simulink model "Exercise1"  (R2024b)
settings: Solver=VariableStepAuto  StartTime=0.0  StopTime=seconds(missionduration)  FixedStep=1  MaxStep=5  RelTol=0.5e-5  AbsTol=1e-5
undefined symbols (not defined in the file): IAU, juliandate, missionstartdate, targetAmazon, targetNO
libraries: aerolibtransform2 x3, aerolibguid x2, aerolibsatdyn x1, aerolibutil x1
settings Model: Creator=The MathWorks, Inc.  LastModifiedBy=jbrault
settings SolverCC: MaxConsecutiveMinStep=10  AutoInsertRateTranBlk=on  DecoupledContinuousIntegration=on  MinimalZcImpactIntegration=on  MaxZcPerStep=1
settings DataIOCC: DatasetSignalFormat=timetable  LoggingIntervals=[0, inf]
settings DebuggingCC: ReadBeforeWriteMsg=DisableAll  WriteAfterWriteMsg=DisableAll  WriteAfterReadMsg=DisableAll  MultiTaskDSMMsg=none  UnconnectedInputMsg=warning  UnconnectedOutputMsg=warning  UnconnectedLineMsg=warning
settings ModelReferenceCC: UpdateModelReferenceTargets=IfOutOfDate  EnableRefExpFcnMdlSchedulingChecks=on
settings SFSimCC: SFSimEcho=off
settings RTWCC: GPUComputeCapability=3.5  DLArmComputeVersion=19.05

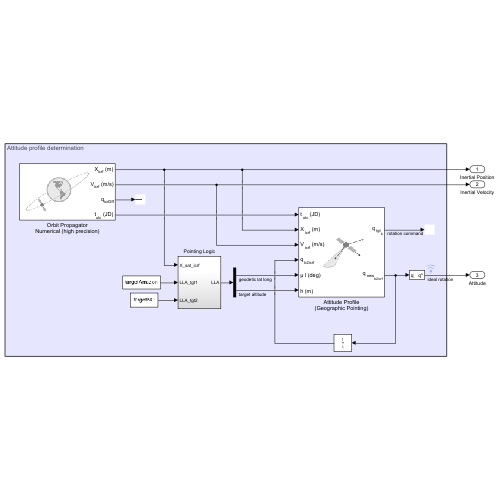
[thumbnail: Simulink's stored preview of the top-level diagram]
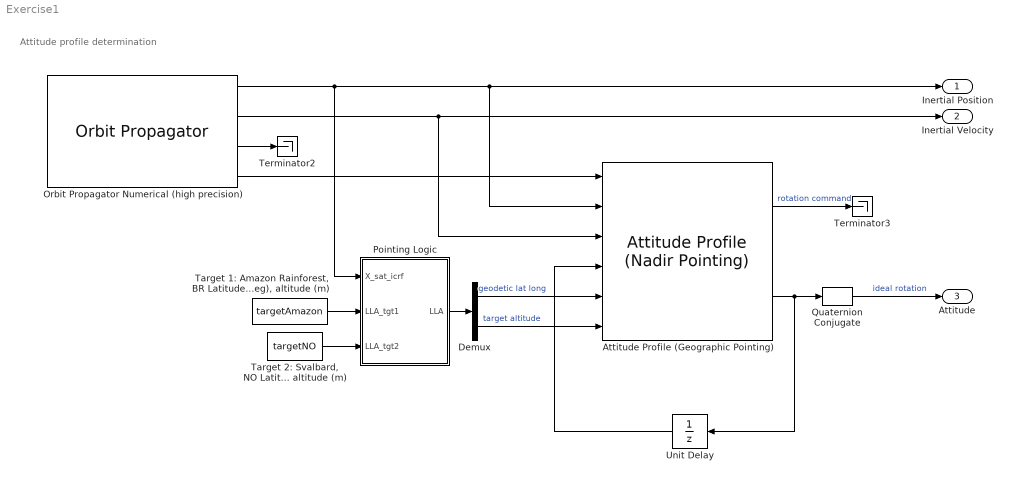
== system Exercise1 ==
  note: Attitude profile determination
  Attitude Profile (Geographic Pointing) : aerolibsatdyn/Attitude Profile (Nadir Pointing)  outputError=on  outputFinalAttitude=on  portFrame=ICRF  pointingMode=Point at LatLonAlt  celestialTarget=Sun  tunablePointing=off  primaryAlignmentSrc=Dialog  primaryAlignment=[0 0 1]  secondaryAlignmentSrc=Dialog  secondaryAlignment=[1 0 0]  constraintFrame=LVLH  primaryConstraintSrc=Dialog  primaryConstraint=[1 0 0]  secondaryConstraintSrc=Dialog  secondaryConstraint=[0 1 0]
  Demux : Demux  Outputs=[2 1]
  Orbit Propagator Numerical (high precision) : OrbitPropagator  propagator=Numerical (high precision)  startDate=juliandate(missionstartdate)  semiMajorAxis=7200000  eccentricity=0.05  inclination=70  raan=215  argPeriapsis=0  trueAnomaly=200  inertialPosition=[3649700.0 3308200.0 -4676600.0]  inertialVelocity=[-2750.8 6666.4 2573.4]  fixedPosition=[-4142689.0 -2676864.7 -4669861.6]  fixedVelocity=[1452.7 -6720.7 2568.1]  customR=3396200  customMu=4.305e13  customJ2=1.0826269e-03  customOmega=4.06125949e-3  outputTransform=on
  Pointing Logic : Subsystem
  Quaternion Conjugate : aerolibutil/Quaternion Conjugate
  "Target 1: Amazon Rainforest, BR Latitude (deg), Longitude (deg), altitude (m)" : Constant  Value=targetAmazon
  "Target 2: Svalbard, NO Latitude (deg), Longitude (deg), altitude (m)" : Constant  Value=targetNO
  Terminator2 : Terminator
  Terminator3 : Terminator
  Unit Delay : UnitDelay  InitialCondition=[1 0 0 0]  SampleTime=-1  HasFrameUpgradeWarning=on
  Inertial Position : Outport
  Inertial Velocity : Outport  Port=2
  Attitude : Outport  Port=3
  wires:
  Orbit Propagator Numerical (high precision)/2 -> Inertial Velocity/1, Attitude Profile (Geographic Pointing)/3
  Orbit Propagator Numerical (high precision)/1 -> Pointing Logic/1(X_sat_icrf), Inertial Position/1, Attitude Profile (Geographic Pointing)/2
  Demux/1 -> Attitude Profile (Geographic Pointing)/5  "geodetic lat long"
  Demux/2 -> Attitude Profile (Geographic Pointing)/6  "target altitude"
  Pointing Logic/1(LLA) -> Demux/1
  "Target 1: Amazon Rainforest, BR Latitude (deg), Longitude (deg), altitude (m)"/1 -> Pointing Logic/2(LLA_tgt1)
  "Target 2: Svalbard, NO Latitude (deg), Longitude (deg), altitude (m)"/1 -> Pointing Logic/3(LLA_tgt2)
  Attitude Profile (Geographic Pointing)/2 -> Quaternion Conjugate/1, Unit Delay/1
  Orbit Propagator Numerical (high precision)/3 -> Terminator2/1
  Orbit Propagator Numerical (high precision)/4 -> Attitude Profile (Geographic Pointing)/1
  Attitude Profile (Geographic Pointing)/1 -> Terminator3/1  "rotation command"
  Unit Delay/1 -> Attitude Profile (Geographic Pointing)/4
  Quaternion Conjugate/1 -> Attitude/1  "ideal rotation"

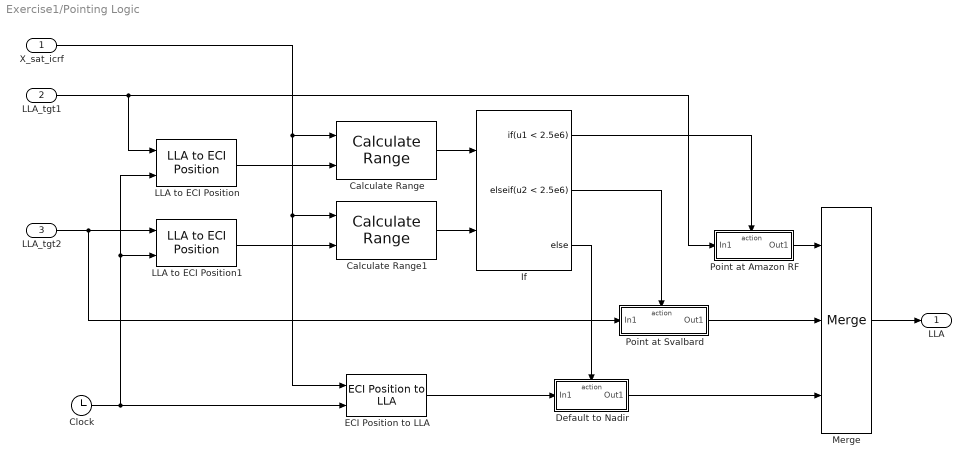
== system Exercise1/Pointing Logic ==
  X_sat_icrf : Inport
  LLA_tgt1 : Inport  Port=2
  LLA_tgt2 : Inport  Port=3
  Calculate Range : aerolibguid/Calculate Range
  Calculate Range1 : aerolibguid/Calculate Range
  Clock : Clock
  Default to Nadir : Subsystem  TreatAsAtomicUnit=on
  ECI Position to LLA : aerolibtransform2/ECI Position to LLA  red=IAU-2000/2006  year=2021  month=January  day=1  hour=12  min=0  sec=0  deltaT=Sec  errorflag=Error  extraparamflag=off  eunits=Metric (MKS)  earthmodel=WGS84  flat=1/298.257223563  eqradius=6378137
      settings: AttributesFormatString=%<red>
  If : If  NumInputs=2  IfExpression=u1 < 2.5e6  ElseIfExpressions=u2 < 2.5e6
  LLA to ECI Position : aerolibtransform2/LLA to ECI Position  red=IAU-2000/2006  year=2021  month=January  day=1  hour=12  min=0  sec=0  deltaT=Sec  errorflag=Error  extraparamflag=off  eunits=Metric (MKS)  earthmodel=WGS84  flat=1/298.257223563  eqradius=6378137
      settings: AttributesFormatString=%<red>
  LLA to ECI Position1 : aerolibtransform2/LLA to ECI Position  red=IAU-2000/2006  year=2021  month=January  day=1  hour=12  min=0  sec=0  deltaT=Sec  errorflag=Error  extraparamflag=off  eunits=Metric (MKS)  earthmodel=WGS84  flat=1/298.257223563  eqradius=6378137
      settings: AttributesFormatString=%<red>
  Merge : Merge  Inputs=3
  Point at Amazon RF : Subsystem  TreatAsAtomicUnit=on
  Point at Svalbard : Subsystem  TreatAsAtomicUnit=on
  LLA : Outport
  wires:
  ECI Position to LLA/1 -> Default to Nadir/1(In1)
  If/3 -> Default to Nadir/Action
  Default to Nadir/1(Out1) -> Merge/3
  Point at Amazon RF/1(Out1) -> Merge/1
  Merge/1 -> LLA/1
  LLA to ECI Position/1 -> Calculate Range/2
  If/1 -> Point at Amazon RF/Action
  If/2 -> Point at Svalbard/Action
  Point at Svalbard/1(Out1) -> Merge/2
  Calculate Range/1 -> If/1
  Calculate Range1/1 -> If/2
  LLA to ECI Position1/1 -> Calculate Range1/2
  LLA_tgt2/1 -> Point at Svalbard/1(In1), LLA to ECI Position1/1
  LLA_tgt1/1 -> Point at Amazon RF/1(In1), LLA to ECI Position/1
  X_sat_icrf/1 -> Calculate Range1/1, ECI Position to LLA/1, Calculate Range/1
  Clock/1 -> LLA to ECI Position/2, LLA to ECI Position1/2, ECI Position to LLA/2

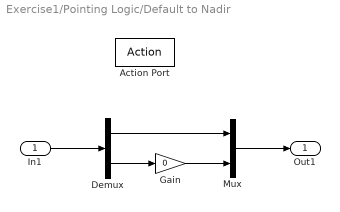
== system Exercise1/Pointing Logic/Default to Nadir ==
  In1 : Inport
  Action Port : ActionPort  ActionPortLabel=else
  Demux : Demux  Outputs=[2, 1]
  Gain : Gain  Gain=0
  Mux : Mux  Inputs=[2, 1]
  Out1 : Outport
  wires:
  In1/1 -> Demux/1
  Demux/1 -> Mux/1
  Demux/2 -> Gain/1
  Gain/1 -> Mux/2
  Mux/1 -> Out1/1

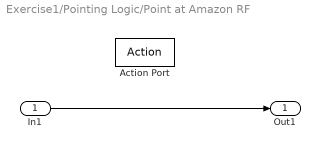
== system Exercise1/Pointing Logic/Point at Amazon RF ==
  In1 : Inport
  Action Port : ActionPort  ActionPortLabel=if(u1 < 2.5e6)
  Out1 : Outport
  wires:
  In1/1 -> Out1/1

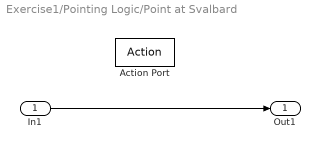
== system Exercise1/Pointing Logic/Point at Svalbard ==
  In1 : Inport
  Action Port : ActionPort  ActionPortLabel=elseif(u2 < 2.5e6)
  Out1 : Outport
  wires:
  In1/1 -> Out1/1
